simulink library "MBDLib_2020"  (R2020b)
settings: Solver=VariableStepAuto  StartTime=0.0  StopTime=10.0  RelTol=1e-3
settings Model: Creator=005274  LastModifiedBy=005274

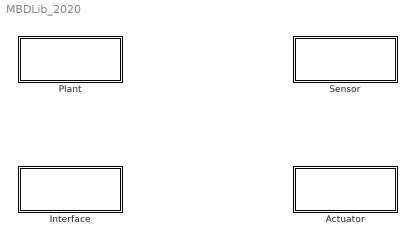
== system MBDLib_2020 ==
  Actuator : Subsystem
  Interface : Subsystem
  Plant : Subsystem
  Sensor : Subsystem

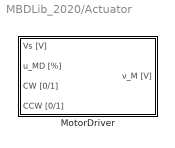
== system MBDLib_2020/Actuator ==
  MotorDriver : Subsystem  mask(MotorDriverModel){}

== system MBDLib_2020/Interface ==

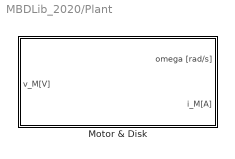
== system MBDLib_2020/Plant ==
  Motor & Disk : Subsystem  mask(DCMotor&DiskModel){R=5.7, L=0.2, J_M=1.1e-4, J_I=1.3e-3, D=6.0e-5, K_tau=7.2e-2, K_e=7.2e-2}
      mask prompts: R "Resistance : R"; L "Inductance : L"; J_M "Moment of Inertia : J_M"; J_I "Moment of Inertia of Load : J_I"; D "Viscus friction : D"; K_tau "Constant torque : K_tau"; K_e "Back electromotive force constant : K_e"

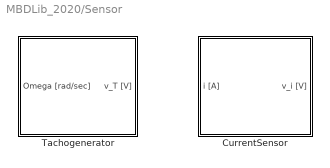
== system MBDLib_2020/Sensor ==
  CurrentSensor : Subsystem  mask(CurrentSensorModel){}
  Tachogenerator : Subsystem  mask(TachoGeneratorModel){}

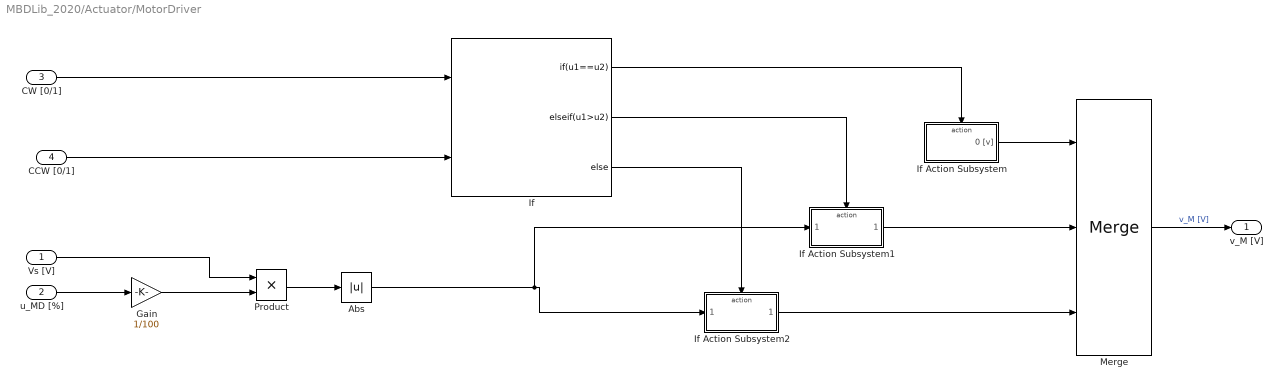
== system MBDLib_2020/Actuator/MotorDriver ==
  Vs [V] : Inport
  u_MD [%] : Inport  Port=2
  CW [0/1] : Inport  Port=3
  CCW [0/1] : Inport  Port=4
  Abs : Abs
  Gain : Gain  Gain=1/100
  If : If  NumInputs=2  IfExpression=u1==u2  ElseIfExpressions=u1>u2
  If Action Subsystem : Subsystem  TreatAsAtomicUnit=on
  If Action Subsystem1 : Subsystem  TreatAsAtomicUnit=on
  If Action Subsystem2 : Subsystem  TreatAsAtomicUnit=on
  Merge : Merge  Inputs=3
  Product : Product
  v_M [V] : Outport
  wires:
  Product/1 -> Abs/1
  Gain/1 -> Product/2
  If Action Subsystem1/1(v_M [V]) -> Merge/2
  If Action Subsystem2/1(-v_M [V]) -> Merge/3
  If/2 -> If Action Subsystem1/Action
  Merge/1 -> v_M [V]/1  "v_M [V]"
  If Action Subsystem/1(0 [v]) -> Merge/1
  If/1 -> If Action Subsystem/Action
  Vs [V]/1 -> Product/1
  If/3 -> If Action Subsystem2/Action
  u_MD [%]/1 -> Gain/1
  Abs/1 -> If Action Subsystem1/1(|v_M| [V]), If Action Subsystem2/1(|v_M| [V])
  CW [0/1]/1 -> If/1
  CCW [0/1]/1 -> If/2

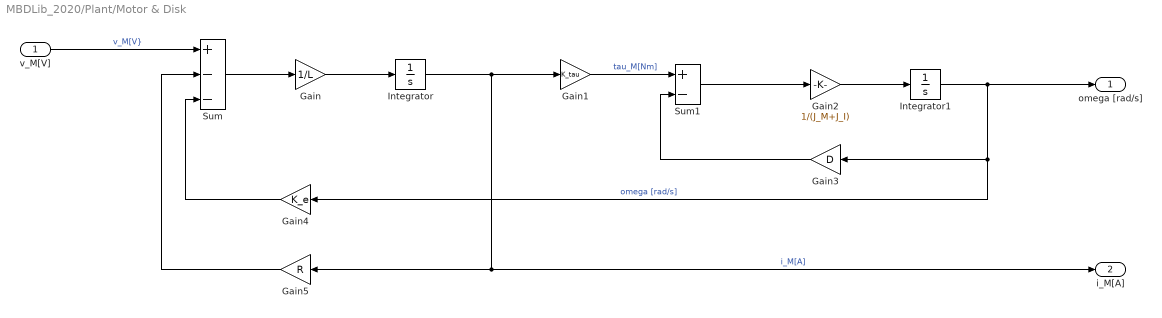
== system MBDLib_2020/Plant/Motor & Disk ==
  v_M[V] : Inport
  Gain : Gain  Gain=1/L
  Gain1 : Gain  Gain=K_tau
  Gain2 : Gain  Gain=1/(J_M+J_I)
  Gain3 : Gain  Gain=D
  Gain4 : Gain  Gain=K_e
  Gain5 : Gain  Gain=R
  Integrator : Integrator
  Integrator1 : Integrator
  Sum : Sum  Inputs=+--
  Sum1 : Sum  Inputs=+-
  "omega [rad/s] " : Outport
  i_M[A] : Outport  Port=2
  wires:
  Integrator1/1 -> "omega [rad/s] "/1, Gain4/1, Gain3/1  "omega [rad/s]"
  Sum/1 -> Gain/1
  Gain/1 -> Integrator/1
  Gain5/1 -> Sum/2
  Gain1/1 -> Sum1/1  "tau_M[Nm]"
  Gain2/1 -> Integrator1/1
  Gain3/1 -> Sum1/2
  Gain4/1 -> Sum/3
  Sum1/1 -> Gain2/1
  v_M[V]/1 -> Sum/1  "v_M[V}"
  Integrator/1 -> Gain1/1, Gain5/1, i_M[A]/1  "i_M[A]"

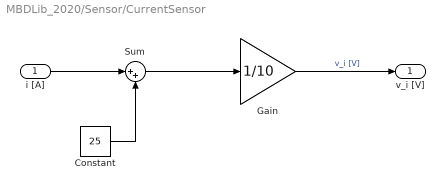
== system MBDLib_2020/Sensor/CurrentSensor ==
  i [A] : Inport
  Constant : Constant  Value=25
  Gain : Gain  Gain=1/10
  Sum : Sum  Inputs=|++
  v_i [V] : Outport
  wires:
  Sum/1 -> Gain/1
  Constant/1 -> Sum/2
  Gain/1 -> v_i [V]/1  "v_i [V]"
  i [A]/1 -> Sum/1

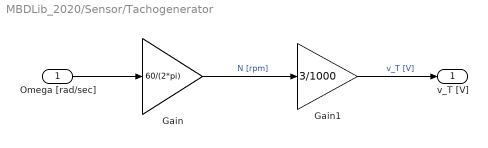
== system MBDLib_2020/Sensor/Tachogenerator ==
  Omega [rad/sec] : Inport
  Gain : Gain  Gain=60/(2*pi)
  Gain1 : Gain  Gain=3/1000
  v_T [V] : Outport
  wires:
  Gain/1 -> Gain1/1  "N [rpm]"
  Omega [rad/sec]/1 -> Gain/1
  Gain1/1 -> v_T [V]/1  "v_T [V]"

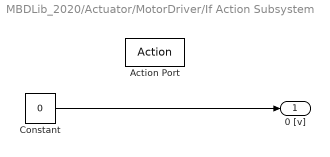
== system MBDLib_2020/Actuator/MotorDriver/If Action Subsystem ==
  Action Port : ActionPort
  Constant : Constant  Value=0
  0 [v] : Outport
  wires:
  Constant/1 -> 0 [v]/1

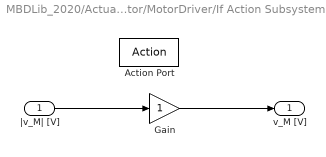
== system MBDLib_2020/Actuator/MotorDriver/If Action Subsystem1 ==
  |v_M| [V] : Inport
  Action Port : ActionPort
  Gain : Gain
  v_M [V] : Outport
  wires:
  |v_M| [V]/1 -> Gain/1
  Gain/1 -> v_M [V]/1

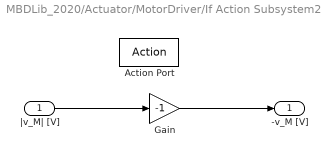
== system MBDLib_2020/Actuator/MotorDriver/If Action Subsystem2 ==
  |v_M| [V] : Inport
  Action Port : ActionPort
  Gain : Gain  Gain=-1
  -v_M [V] : Outport
  wires:
  |v_M| [V]/1 -> Gain/1
  Gain/1 -> -v_M [V]/1
